simulink model "Motorul_de_curent_continuu"  (R2021b)
settings: Solver=VariableStepAuto  StartTime=0.0  StopTime=50  RelTol=1e-3
values from neighbouring files (symbols this model uses):
  A = [-1/Ta -ke/La;km/J 0]    [valori_mcc.m]    (also in valori_sistem_de_incazire_pardoseala.m = [-1/Tp 1/Tp;kp/(kc*Tc) -((1+kp/kc)/Tc)])
  B = [kE/La 0;0 -1/J]    [valori_mcc.m]    (also in valori_sistem_de_incazire_pardoseala.m = [kE/(kp*Tp) 0;0 1/Tc])
  C = [1 0;0 1]    [valori_mcc.m]    (also in valori_sistem_de_incazire_pardoseala.m = [0 1])
  D = [0 0;0 0]    [valori_mcc.m]    (also in valori_sistem_de_incazire_pardoseala.m = [0 0])
  J = 0.0302    [valori_mcc.m]
  kE = 42.85    [valori_mcc.m]    (also in valori_sistem_de_incazire_pardoseala.m = 1000)
  ke = 0.56    [valori_mcc.m]
  km = 0.55    [valori_mcc.m]
  Ra = 5.1    [valori_mcc.m]
  Ta = 0.1    [valori_mcc.m]
  Tm = 0.5    [valori_mcc.m]
settings Model: Creator=alexandra.szedlak-st  LastModifiedBy=alexandra.szedlak-st

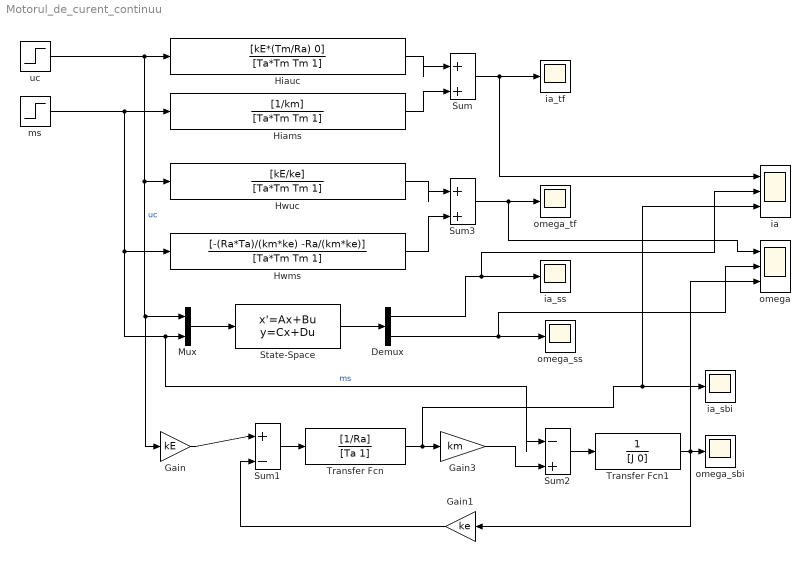
== system Motorul_de_curent_continuu ==
  Demux : Demux  Outputs=2
  Gain : Gain  Gain=kE
  Gain1 : Gain  Gain=ke
  Gain3 : Gain  Gain=km
  Hiams : TransferFcn  Numerator=[1/km]  Denominator=[Ta*Tm Tm 1]
  Hiauc : TransferFcn  Numerator=[kE*(Tm/Ra) 0]  Denominator=[Ta*Tm Tm 1]
  Hwms : TransferFcn  Numerator=[-(Ra*Ta)/(km*ke) -Ra/(km*ke)]  Denominator=[Ta*Tm Tm 1]
  Hwuc : TransferFcn  Numerator=[kE/ke]  Denominator=[Ta*Tm Tm 1]
  Mux : Mux  Inputs=2
  State-Space : StateSpace  A=A  B=B  C=C  D=D  InitialCondition=0
  Sum : Sum  Inputs=|++
  Sum1 : Sum  Inputs=|+-
  Sum2 : Sum  Inputs=|-+
  Sum3 : Sum  Inputs=|++
  Transfer Fcn : TransferFcn  Numerator=[1/Ra]  Denominator=[Ta 1]
  Transfer Fcn1 : TransferFcn  Denominator=[J 0]
  ia : Scope  NumInputPorts=3
  ia_sbi : Scope
  ia_ss : Scope
  ia_tf : Scope
  ms : Step  Time=30  SampleTime=0
  omega : Scope  NumInputPorts=3
  omega_sbi : Scope
  omega_ss : Scope
  omega_tf : Scope
  uc : Step  Time=0  After=3.5  SampleTime=0
  wires:
  uc/1 -> Hwuc/1, Gain/1, Mux/1, Hiauc/1  "uc"
  ms/1 -> Hwms/1, Sum2/1, Mux/2, Hiams/1  "ms"
  Hiauc/1 -> Sum/1
  Hiams/1 -> Sum/2
  Sum/1 -> ia/1, ia_tf/1
  Mux/1 -> State-Space/1
  Sum1/1 -> Transfer Fcn/1
  Transfer Fcn/1 -> ia/3, ia_sbi/1, Gain3/1
  Gain3/1 -> Sum2/2
  Sum2/1 -> Transfer Fcn1/1
  Transfer Fcn1/1 -> omega/3, omega_sbi/1, Gain1/1
  State-Space/1 -> Demux/1
  Hwms/1 -> Sum3/2
  Hwuc/1 -> Sum3/1
  Sum3/1 -> omega/1, omega_tf/1
  Demux/2 -> omega/2, omega_ss/1
  Demux/1 -> ia/2, ia_ss/1
  Gain1/1 -> Sum1/2
  Gain/1 -> Sum1/1
